simulink model "Simulink_MPC_Main"  (R2023b)
settings: Solver=ode1  StartTime=0.0  StopTime=100  FixedStep=SampleTime  MaxStep=0.01  RelTol=1e-3  EnableMultiTasking=on
values from neighbouring files (symbols this model uses):
  Delay = 3    [Prepare_MPC_005.m]
  FilterDer0 = [8.542800360484532896e-02 ... (first row only)    [Prepare_MPC_005.m]
  FilterDer1 = [2.939212680227305530e+00 ... (first row only)    [Prepare_MPC_005.m]
  SampleTime = 0.05    [Prepare_MPC_005.m]
undefined symbols (not defined in the file or in its folder): GetPosition, length_trajectory_s, poly_approx_trajectory, UpdateBoard
libraries: sldrtlib x1
(part 1 of 2)
settings Model: Creator=jgillis  LastModifiedBy=heib
settings SolverCC: ConcurrentTasks=on  AlgebraicLoopSolver=TrustRegion  PositivePriorityOrder=on  AutoInsertRateTranBlk=on
settings DataIOCC: LimitDataPoints=on  SaveFormat=Array  ReturnWorkspaceOutputs=off
settings OptimizationCC: BlockReduction=off  OptimizeBlockIOStorage=off
settings DebuggingCC: SolverPrmCheckMsg=warning  TasksWithSamePriorityMsg=none  UnconnectedInputMsg=warning  UnconnectedOutputMsg=warning  UnconnectedLineMsg=warning  SFUnexpectedBacktrackingDiag=warning  SFNoUnconditionalDefaultTransitionDiag=warning  SFExecutionAtInitializationDiag=none  ArithmeticOperatorsInVariantConditions=warning
settings HardwareCC: ProdBitPerLong=64  ProdHWDeviceType=Intel->x86-64 (Linux 64)
settings ModelReferenceCC: EnableRefExpFcnMdlSchedulingChecks=on  PropagateSignalLabelsOutOfModel=off
settings SFSimCC: SimUseLocalCustomCode=off  CustomCodeUndefinedFunction=UseInterfaceOnly
settings RTWCC: Description=Simulink Desktop Real-Time  SystemTargetFile=sldrt.tlc  TemplateMakefile=sldrt.tmf  RTWUseLocalCustomCode=off  CustomLibrary=Casadi\casadi.lib  BuildConfiguration=Faster Runs  RTWCompilerOptimization=on
settings CodeAppCC: MaxIdLength=95  StateflowObjectComments=on
settings SimulinkDesktopRealTimeCC: TargetLibSuffix=_sldrt.a  TargetPreCompLibLocation=/home/heib/Documents/Matlab23b/toolbox/sldrt/lib/glnxa64
settings ConfigComp: CovMetricSettings=dw  CovSaveCumulativeToWorkspaceVar=on  CovSaveSingleToWorkspaceVar=on  CovExternalEMLEnable=off  CovSFcnEnable=off

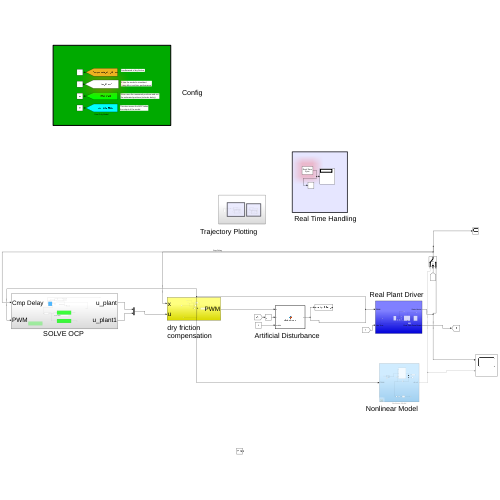
[thumbnail: Simulink's stored preview of the top-level diagram]
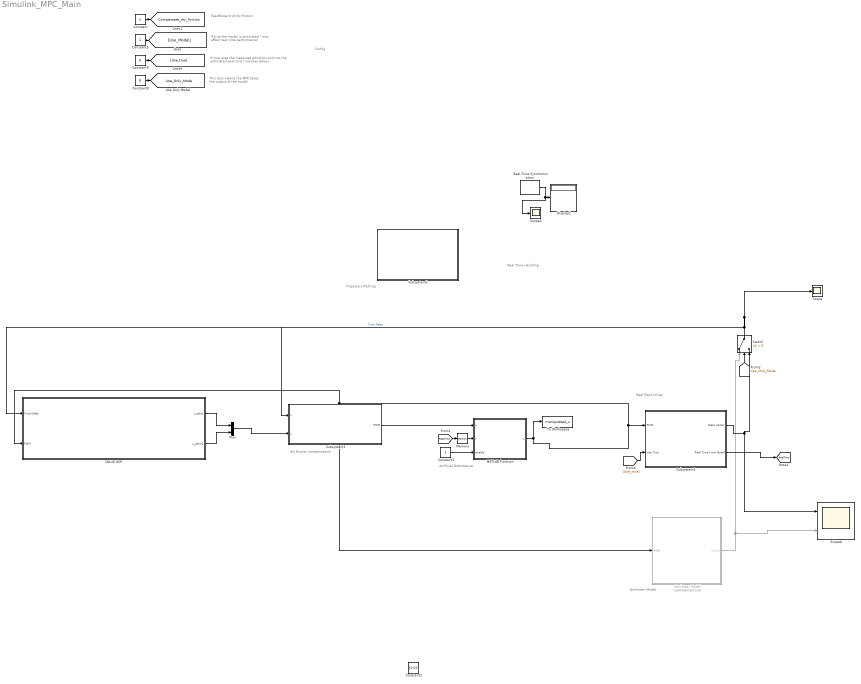
== system Simulink_MPC_Main ==
  note: dry friction compensation
  note: This also means the MPC takes
      | the output of the model
  note: If true the model is simulated
      | ! may affect real time performance!
  note: If true uses the messured positions and not
      | the estimated positions (includes delay).
  note: Feedforward of dry friction
  note: Nonlinear Model
  note: Real Plant Driver
  note: Real Time Handling
  note: Trajectory Plotting
  note: Config
  note: Artificial Disturbance
  Constant : Constant
  Constant1 : Constant
  Constant2 : Constant  Value=[0 0]'
  Constant5 : Constant
  Constant8 : Constant  Value=0
  Constant9 : Constant  Value=0
  Display2 : Display
  MATLAB Function : MATLAB Function  TreatAsAtomicUnit=on
  Memory : Memory
  Mux : Mux  Inputs=2
  Nonlinear Model : Subsystem  Commented=on
  Real-Time Synchronization : sldrtlib/Real-Time Synchronization  SampleTime=SampleTime  MaxMissedTicks=200  ShowMissedTicks=on  YieldWhenWaiting=off
  "SOLVE OCP " : Subsystem
  Scope : Scope
  Scope3 : Scope
  Scope6 : Scope  NumInputPorts=2
  Subsystem1 : Subsystem
  Subsystem2 : Subsystem
  Subsystem3 : Subsystem
  Switch : Switch  Criteria=u2 > Threshold  SaturateOnIntegerOverflow=off  InputSameDT=off
  To Workspace : ToWorkspace  VariableName=manipulated_u  SaveFormat=Timeseries  SampleTime=-1
  tag scope: Compensate_dry_friction=global, RealTime=global, Use_Only_Mode=global
  wires:
  Real-Time Synchronization/1 -> Scope3/1, Display2/1
  MATLAB Function/1(u) -> To Workspace/1, Nonlinear Model/1(PWM), "SOLVE OCP "/2(PWM), Subsystem1/1(PWM)
  Constant8/1 -> [Use_Only_Mode]
  Constant9/1 -> [Use_true]
  Constant5/1 -> [Use_Model]
  Constant/1 -> [Compensate_dry_friction]
  [Use_Only_Mode] -> Switch/2
  Nonlinear Model/1(x0 z-1) -> Scope6/2, Switch/1
  [Use_true] -> Subsystem1/2(Use True)
  Switch/1 -> Scope/1, "SOLVE OCP "/1(Cmp Delay), Subsystem3/1(x)  "Cmp Delay"
  Subsystem1/2(Real Time From Board) -> [RealTime]
  "SOLVE OCP "/1(u_plant) -> Mux/1
  "SOLVE OCP "/2(u_plant1) -> Mux/2
  Subsystem1/1(State Vector) -> Switch/3, Scope6/1
  Mux/1 -> Subsystem3/2(u)
  Subsystem3/1(PWM) -> MATLAB Function/1("u ")
  [RealTime] -> Memory/1
  Memory/1 -> MATLAB Function/2(t)
  Constant1/1 -> MATLAB Function/3(enable)

== system Simulink_MPC_Main/Nonlinear Model ==
  PWM : Inport
  Constant : Constant  Value=0
  Constant1 : Constant  Value=SampleTime
  Demux : Demux  Outputs=2
  MATLAB Function3 : MATLAB Function  TreatAsAtomicUnit=on
  MATLAB Function4 : MATLAB Function  TreatAsAtomicUnit=on
  Memory : Memory  InitialCondition=[GetPosition;zeros(5,1)]'  InheritSampleTime=on
  Memory1 : Memory  InitialCondition=[GetPosition;zeros(5,1)]'  InheritSampleTime=on
  Memory2 : Memory  InitialCondition=[GetPosition;zeros(5,1)]'  InheritSampleTime=on
  Mux : Mux  Inputs=3
  Scope2 : Scope
  To Workspace2 : ToWorkspace  VariableName=Rk4_results  SaveFormat=Timeseries  SampleTime=-1
  x0 z-1 : Outport
  wires:
  MATLAB Function4/1(x_end) -> To Workspace2/1, Memory/1, Scope2/1
  Memory/1 -> Memory1/1, MATLAB Function4/1(x_in)
  PWM/1 -> Demux/1
  Demux/1 -> Mux/1
  Demux/2 -> Mux/2
  Constant/1 -> Mux/3
  Mux/1 -> MATLAB Function4/2(PWM)
  Memory1/1 -> Memory2/1
  Memory2/1 -> MATLAB Function3/1(x)
  Constant1/1 -> MATLAB Function4/3(SampleTime)
  MATLAB Function3/1(current) -> x0 z-1/1

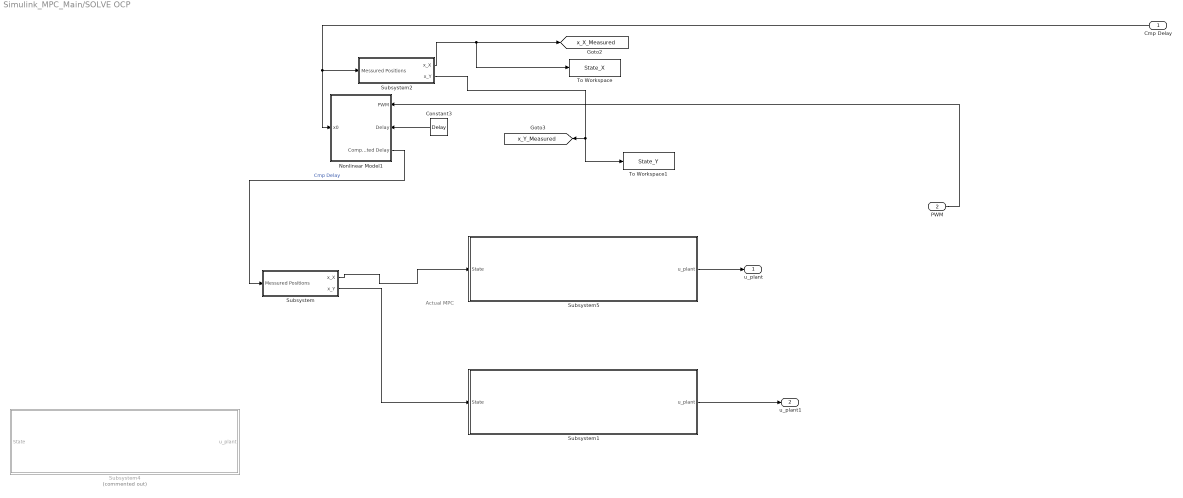
== system Simulink_MPC_Main/SOLVE OCP  ==
  note: Actual MPC
  Cmp Delay : Inport
  PWM : Inport  Port=2
  Constant3 : Constant  Value=Delay
  Nonlinear Model1 : Subsystem
      settings: PortSchema="{\"entries\":[{\"content\":{\"sides\":[{\"content\":{\"connectorIds\":[\"In1\"]},\"type\":\"ConnectorPlacement.EquallySpacedRectSide\",\"uuid\":\"38cfd3d7-56a6-4f45-9bca-759458190eeb\"},{\"content\":{\"connectorIds\":[\"In2\",\"In3\",\"Out1\"],\"side\":\"RIGHT\"},\"type\":\"ConnectorPlacement.EquallySpacedRectSide\",\"uuid\":\"8f579a40-73f0-4433-ae4d-9a35b6fc4d2d\"},{\"content\":{\"side\":\"TOP\"},\"type\":\"ConnectorPlacement.EquallySpacedRectSide\",\"uuid\":\"6933b4ac-f36e-403d-9ee4-935888590ea9\"}]},\"type\":\"ConnectorPlacement.EquallySpacedConnector\",\"uuid\":\"01f2f68f-8bb5-4722-9573-e5e42a50f642\"}],\"packageUris\":[\"http://schema.mathworks.com/mf0/Connector/R2020b\"],\"version\":\"1.0\"}"
  Subsystem : Subsystem
  Subsystem1 : Subsystem
  Subsystem2 : Subsystem
  Subsystem4 : Subsystem  Commented=on
  Subsystem5 : Subsystem
  To Workspace : ToWorkspace  VariableName=State_X  SaveFormat=Timeseries  SampleTime=-1
  To Workspace1 : ToWorkspace  VariableName=State_Y  SaveFormat=Timeseries  SampleTime=-1
  u_plant : Outport
  u_plant1 : Outport  Port=2
  tag scope: x_X_Measured=global, x_Y_Measured=global
  wires:
  Nonlinear Model1/1(Compensated Delay) -> Subsystem/1(Messured Positions)  "Cmp Delay"
  Cmp Delay/1 -> Subsystem2/1(Messured Positions), Nonlinear Model1/1(x0)
  Constant3/1 -> Nonlinear Model1/3(Delay)
  Subsystem1/1(u_plant) -> u_plant1/1
  PWM/1 -> Nonlinear Model1/2(PWM)
  Subsystem5/1(u_plant) -> u_plant/1
  Subsystem/1(x_X) -> Subsystem5/1(State)
  Subsystem/2(x_Y) -> Subsystem1/1(State)
  Subsystem2/1(x_X) -> To Workspace/1, [x_X_Measured]
  Subsystem2/2(x_Y) -> To Workspace1/1, [x_Y_Measured]

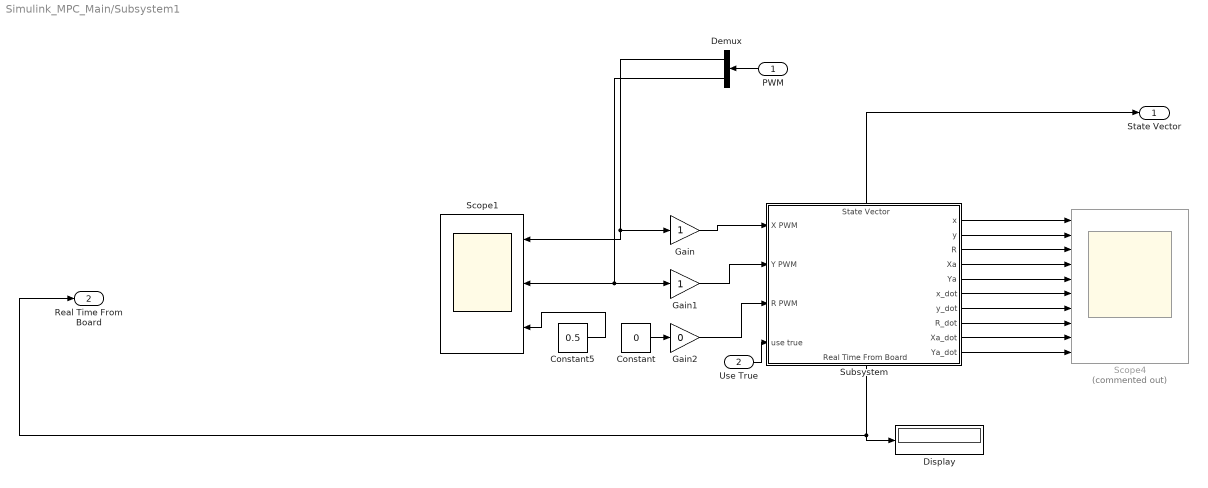
== system Simulink_MPC_Main/Subsystem1 ==
  PWM : Inport
  Use True : Inport  Port=2
  Constant : Constant  Value=0
  Constant5 : Constant  Value=0.5
  Demux : Demux  Outputs=2
  Display : Display
  Gain : Gain
  Gain1 : Gain
  Gain2 : Gain  Gain=0
  Scope1 : Scope  NumInputPorts=3
  Scope4 : Scope  Commented=on  NumInputPorts=10
  Subsystem : Subsystem  StopFcn=UpdateBoard([0 0 0])
      settings: PortSchema="{\"entries\":[{\"content\":{\"sides\":[{\"content\":{\"connectorIds\":[\"In1\",\"In2\",\"In3\",\"In4\"]},\"type\":\"ConnectorPlacement.EquallySpacedRectSide\",\"uuid\":\"9c191be3-a45d-4bde-908f-a93b32fc7100\"},{\"content\":{\"connectorIds\":[\"Out1\",\"Out2\",\"Out3\",\"Out4\",\"Out5\",\"Out6\",\"Out7\",\"Out8\",\"Out9\",\"Out10\"],\"side\":\"RIGHT\"},\"type\":\"ConnectorPlacement.EquallySpacedRectSide\",\"uuid\":\"786ae7fd-3fdd-4e4f-b32e-e8a30c9c90df\"},{\"content\":{\"connectorIds\":[\"Out12\"],\"side\":\"TOP\"},\"type\":\"ConnectorPlacement.EquallySpacedRectSide\",\"uuid\":\"660763ff-34dc-4c5b-8e93-3606a4818ae8\"},{\"content\":{\"connectorIds\":[\"Out11\"],\"side\":\"BOTTOM\"},\"type\":\"ConnectorPlacement.EquallySpacedRectSide\",\"uuid\":\"dc7e5dc1-ad21-4d2b-aff3-6d4be469e1a4\"}]},\"type\":\"ConnectorPlacement.EquallySpacedConnector\",\"uuid\":\"7e886ff6-44b8-4e6d-bf22-6606d53ee007\"}],\"packageUris\":[\"http://schema.mathworks.com/mf0/Connector/R2020b\"],\"version\":\"1.0\"}"
  State Vector : Outport
  Real Time From Board : Outport  Port=2
  wires:
  Subsystem/4(Xa) -> Scope4/4
  Subsystem/1(x) -> Scope4/1
  Subsystem/9(Xa_dot) -> Scope4/9
  Subsystem/10(Ya_dot) -> Scope4/10
  Subsystem/3(R) -> Scope4/3
  Subsystem/8(R_dot) -> Scope4/8
  Subsystem/7(y_dot) -> Scope4/7
  Subsystem/11(Real Time From Board) -> Real Time From Board/1, Display/1
  Subsystem/5(Ya) -> Scope4/5
  Subsystem/12(State Vector) -> State Vector/1
  Constant5/1 -> Scope1/3
  Gain/1 -> Subsystem/1(X PWM)
  Subsystem/2(y) -> Scope4/2
  Gain2/1 -> Subsystem/3(R PWM)
  Subsystem/6(x_dot) -> Scope4/6
  Demux/1 -> Scope1/1, Gain/1
  Demux/2 -> Gain1/1, Scope1/2
  Constant/1 -> Gain2/1
  Gain1/1 -> Subsystem/2(Y PWM)
  PWM/1 -> Demux/1
  Use True/1 -> Subsystem/4(use true)

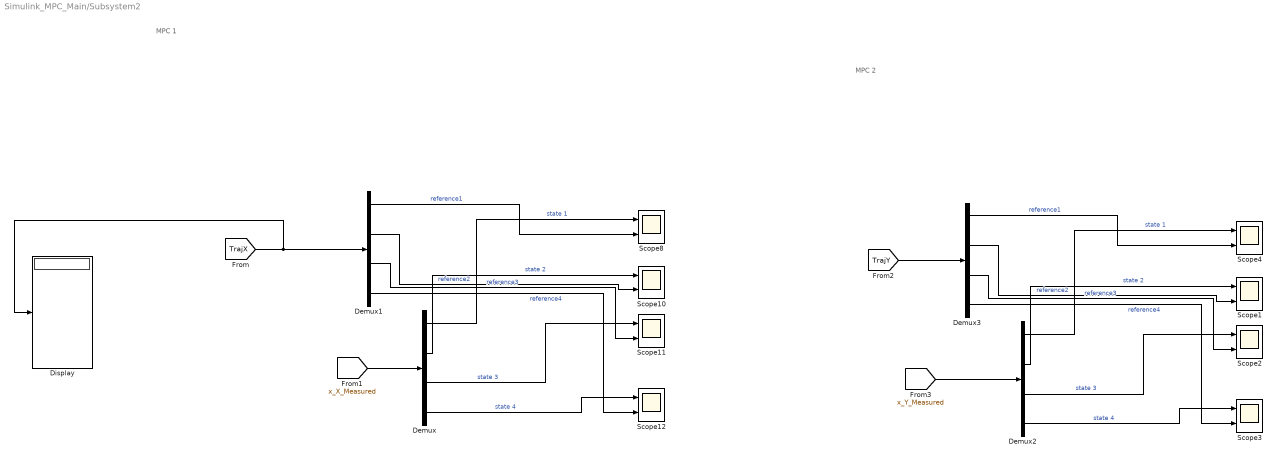
== system Simulink_MPC_Main/Subsystem2 ==
  note: MPC 1
  note: MPC 2
  Demux{,1..3} (4 alike) : Demux
  Display : Display
  Scope{1..4,8,10..12} (8 alike) : Scope  NumInputPorts=2
  wires:
  [x_X_Measured] -> Demux/1
  Demux/1 -> Scope8/1  "state 1"
  Demux/2 -> Scope10/1  "state 2"
  Demux/3 -> Scope11/1  "state 3"
  Demux/4 -> Scope12/1  "state 4"
  Demux1/4 -> Scope12/2  "reference4"
  Demux1/3 -> Scope11/2  "reference3"
  Demux1/2 -> Scope10/2  "reference2"
  Demux1/1 -> Scope8/2  "reference1"
  Demux2/4 -> Scope3/1  "state 4"
  [x_Y_Measured] -> Demux2/1
  Demux2/2 -> Scope1/1  "state 2"
  Demux3/3 -> Scope2/2  "reference3"
  Demux3/2 -> Scope1/2  "reference2"
  Demux3/4 -> Scope3/2  "reference4"
  Demux2/3 -> Scope2/1  "state 3"
  Demux2/1 -> Scope4/1  "state 1"
  Demux3/1 -> Scope4/2  "reference1"
  [TrajX] -> Demux1/1, Display/1
  [TrajY] -> Demux3/1

== system Simulink_MPC_Main/Subsystem3 ==
  x : Inport
  u : Inport  Port=2
  Scope : Scope  NumInputPorts=2
  Switch : Switch  Criteria=u2 > Threshold  SaturateOnIntegerOverflow=off  InputSameDT=off
  To Workspace3 : ToWorkspace  VariableName=PWM_toPlant  SaveFormat=Timeseries  SampleTime=-1
  dry_friction_compensation : MATLAB Function  TreatAsAtomicUnit=on
  PWM : Outport
  wires:
  x/1 -> dry_friction_compensation/1(x)
  dry_friction_compensation/1(u_compensated) -> Switch/1
  u/1 -> Scope/1, dry_friction_compensation/2(u), Switch/3
  Switch/1 -> Scope/2, To Workspace3/1, PWM/1
  [Compensate_dry_friction] -> Switch/2

== system Simulink_MPC_Main/SOLVE OCP /Nonlinear Model1 ==
  x0 : Inport
  PWM : Inport  Port=2
  Delay : Inport  Port=3
  Constant : Constant  Value=0
  Constant1 : Constant  Value=SampleTime
  Demux : Demux  Outputs=2
  MATLAB Function : MATLAB Function  TreatAsAtomicUnit=on
  MATLAB Function11 : MATLAB Function  TreatAsAtomicUnit=on
  MATLAB Function4 : MATLAB Function  TreatAsAtomicUnit=on
  Mux : Mux  Inputs=3
  Scope : Scope  NumInputPorts=2
  Compensated Delay : Outport
  wires:
  x0/1 -> Scope/2, MATLAB Function4/1(x_in)  "measured"
  PWM/1 -> Demux/1
  Demux/1 -> Mux/1
  Demux/2 -> Mux/2
  Constant/1 -> Mux/3
  Constant1/1 -> MATLAB Function4/3(SampleTime)
  Delay/1 -> MATLAB Function4/4(Delay)
  MATLAB Function4/1(x_end) -> Scope/1, MATLAB Function/1(x)
  Mux/1 -> MATLAB Function11/1(u)
  MATLAB Function11/1(y) -> MATLAB Function4/2(PWM)
  MATLAB Function/1(x_bound) -> Compensated Delay/1

== system Simulink_MPC_Main/SOLVE OCP /Subsystem ==
  note: Integrator Logic
      | Gemessene Position kommt von Plant
      | und Integral anteil fehler kommt con MPC
  Messured Positions : Inport
  Delete L : MATLAB Function  TreatAsAtomicUnit=on
  MATLAB Function10 : MATLAB Function  TreatAsAtomicUnit=on
  Scope : Scope  Commented=on
  To Workspace5 : ToWorkspace  VariableName=x0_out  SaveFormat=Structure With Time  SampleTime=-1
  x_X : Outport
  x_Y : Outport  Port=2
  wires:
  MATLAB Function10/1(x_X) -> x_X/1, To Workspace5/1
  Messured Positions/1 -> Delete L/1(x10)
  Delete L/1(x_8) -> Scope/1, MATLAB Function10/1(x_18)
  MATLAB Function10/2(x_Y) -> x_Y/1

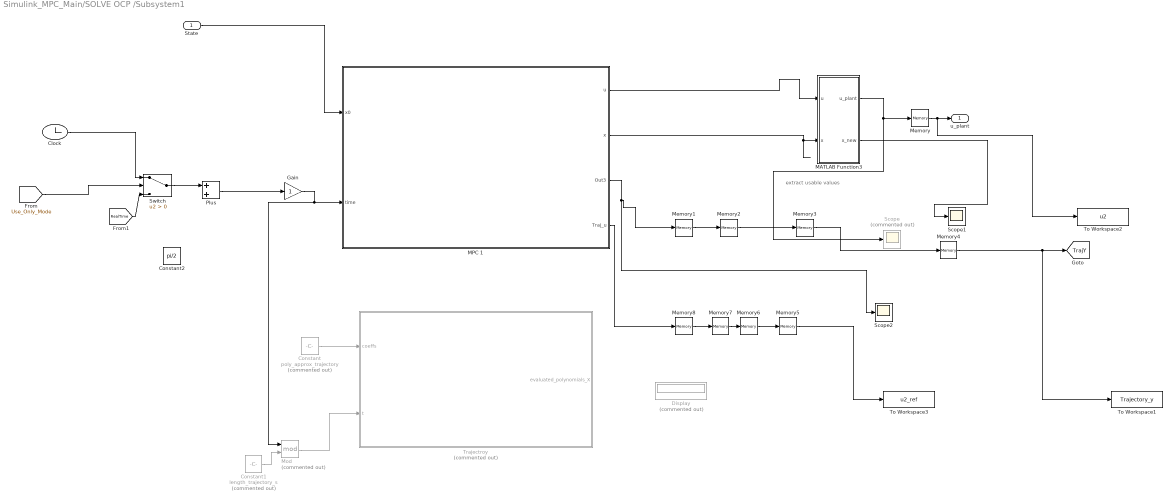
== system Simulink_MPC_Main/SOLVE OCP /Subsystem1 ==
  note: extract usable values
  State : Inport
  Clock : Clock
  Constant : Constant  Commented=on  Value=poly_approx_trajectory
  Constant1 : Constant  Commented=on  Value=length_trajectory_s
  Constant2 : Constant  Value=pi/2
  Display : Display  Commented=on
  Gain : Gain
  MATLAB Function3 : MATLAB Function  TreatAsAtomicUnit=on
  MPC 1 : Subsystem
  Memory{,1..8} (9 alike) : Memory
  Mod : Math  Commented=on  Operator=mod
  Plus : Sum
  Scope : Scope  Commented=on
  Scope1 : Scope
  Scope2 : Scope
  Switch : Switch  Criteria=u2 > Threshold  SaturateOnIntegerOverflow=off  InputSameDT=off
  To Workspace1 : ToWorkspace  VariableName=Trajectory_y  SaveFormat=Timeseries  SampleTime=-1
  To Workspace2 : ToWorkspace  VariableName=u2  SaveFormat=Timeseries  SampleTime=-1
  To Workspace3 : ToWorkspace  VariableName=u2_ref  SaveFormat=Timeseries  SampleTime=-1
  Trajectroy : MATLAB Function  Commented=on  TreatAsAtomicUnit=on
  u_plant : Outport
  tag scope: TrajY=global
  wires:
  MPC 1/2(x) -> MATLAB Function3/2(x)
  MPC 1/1(u) -> MATLAB Function3/1(u)
  Switch/1 -> Plus/1
  MATLAB Function3/1(u_plant) -> Scope/1, Memory/1
  Gain/1 -> MPC 1/2(time), Mod/1
  State/1 -> MPC 1/1(x0)
  Memory/1 -> To Workspace2/1, u_plant/1
  [Use_Only_Mode] -> Switch/2
  Clock/1 -> Switch/1
  [RealTime] -> Switch/3
  MATLAB Function3/2(x_new) -> Scope1/1
  Constant/1 -> Trajectroy/1(coeffs)
  Constant1/1 -> Mod/2
  Mod/1 -> Trajectroy/2(t)
  MPC 1/4(Traj_u) -> Memory8/1
  Plus/1 -> Gain/1
  Memory1/1 -> Memory2/1
  Memory2/1 -> Memory3/1
  Memory3/1 -> Memory4/1
  Memory4/1 -> To Workspace1/1, [TrajY]
  MPC 1/3(Out3) -> Memory1/1, Scope2/1
  Memory7/1 -> Memory6/1
  Memory5/1 -> To Workspace3/1
  Memory8/1 -> Memory7/1
  Memory6/1 -> Memory5/1

== system Simulink_MPC_Main/SOLVE OCP /Subsystem2 ==
  note: Integrator Logic
      | Gemessene Position kommt von Plant
      | und Integral anteil fehler kommt con MPC
  Messured Positions : Inport
  Delete L : MATLAB Function  TreatAsAtomicUnit=on
  MATLAB Function10 : MATLAB Function  TreatAsAtomicUnit=on
  Scope : Scope  Commented=on
  x_X : Outport
  x_Y : Outport  Port=2
  wires:
  MATLAB Function10/1(x_X) -> x_X/1
  Delete L/1(x_8) -> Scope/1, MATLAB Function10/1(x_18)
  MATLAB Function10/2(x_Y) -> x_Y/1
  Messured Positions/1 -> Delete L/1(x10)

== system Simulink_MPC_Main/SOLVE OCP /Subsystem4 ==
  note: extract usable values
  State : Inport
  Clock : Clock
  Constant : Constant  Value=3*pi/2
  Display : Display
  Gain : Gain
  MATLAB Function3 : MATLAB Function  TreatAsAtomicUnit=on
  MPC 1 : Subsystem
  Memory : Memory
  Plus : Sum
  Scope : Scope
  Scope1 : Scope
  u_plant : Outport
  tag scope: TrajY=global
  wires:
  MATLAB Function3/1(u_plant) -> Memory/1, Scope/1
  MPC 1/2(x) -> MATLAB Function3/2(x)
  MPC 1/1(u) -> MATLAB Function3/1(u), Display/1
  Clock/1 -> Plus/1
  Memory/1 -> u_plant/1
  MPC 1/3(Out3) -> [TrajY]
  Gain/1 -> MPC 1/2(time)
  State/1 -> Scope1/1, MPC 1/1(x0)
  Constant/1 -> Plus/2
  Plus/1 -> Gain/1

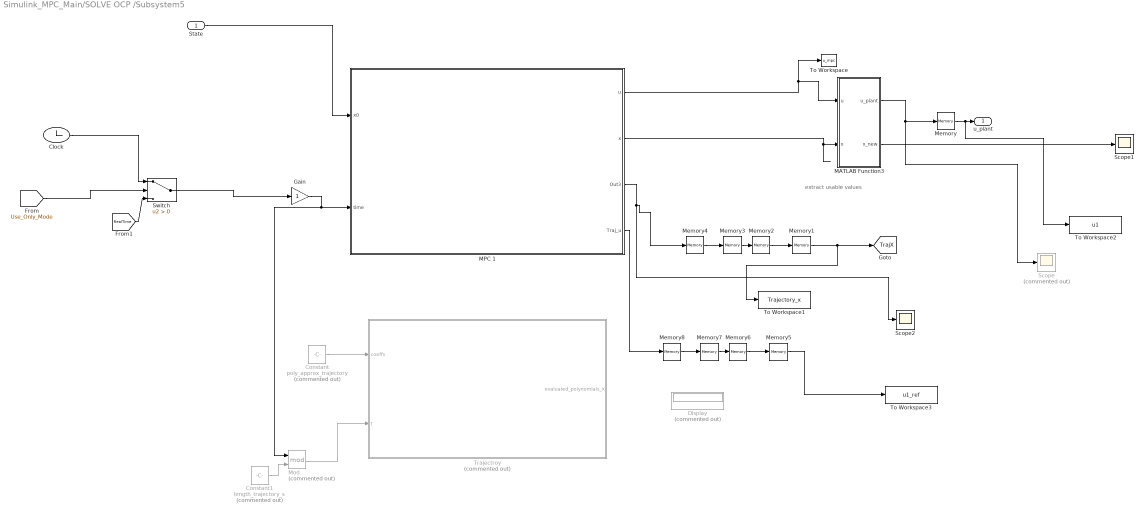
== system Simulink_MPC_Main/SOLVE OCP /Subsystem5 ==
  note: extract usable values
  State : Inport
  Clock : Clock
  Constant : Constant  Commented=on  Value=poly_approx_trajectory
  Constant1 : Constant  Commented=on  Value=length_trajectory_s
  Display : Display  Commented=on
  Gain : Gain
  MATLAB Function3 : MATLAB Function  TreatAsAtomicUnit=on
  MPC 1 : Subsystem
  Memory{,1..8} (9 alike) : Memory
  Mod : Math  Commented=on  Operator=mod
  Scope : Scope  Commented=on
  Scope1 : Scope
  Scope2 : Scope
  Switch : Switch  Criteria=u2 > Threshold  SaturateOnIntegerOverflow=off  InputSameDT=off
  To Workspace : ToWorkspace  VariableName=u_mpc  SaveFormat=Timeseries  SampleTime=-1
  To Workspace1 : ToWorkspace  VariableName=Trajectory_x  SaveFormat=Timeseries  SampleTime=-1
  To Workspace2 : ToWorkspace  VariableName=u1  SaveFormat=Timeseries  SampleTime=-1
  To Workspace3 : ToWorkspace  VariableName=u1_ref  SaveFormat=Timeseries  SampleTime=-1
  Trajectroy : MATLAB Function  Commented=on  TreatAsAtomicUnit=on
  u_plant : Outport
  tag scope: TrajX=global
  wires:
  MPC 1/2(x) -> MATLAB Function3/2(x)
  MPC 1/1(u) -> MATLAB Function3/1(u), To Workspace/1
  Switch/1 -> Gain/1
  Gain/1 -> MPC 1/2(time), Mod/1
  State/1 -> MPC 1/1(x0)
  MATLAB Function3/1(u_plant) -> Memory/1, Scope/1
  [Use_Only_Mode] -> Switch/2
  Clock/1 -> Switch/1
  [RealTime] -> Switch/3
  MPC 1/3(Out3) -> Memory4/1, Scope2/1
  Constant/1 -> Trajectroy/1(coeffs)
  Constant1/1 -> Mod/2
  Mod/1 -> Trajectroy/2(t)
  MATLAB Function3/2(x_new) -> Scope1/1
  Memory/1 -> To Workspace2/1, u_plant/1
  MPC 1/4(Traj_u) -> Memory8/1
  Memory1/1 -> To Workspace1/1, [TrajX]
  Memory2/1 -> Memory1/1
  Memory3/1 -> Memory2/1
  Memory4/1 -> Memory3/1
  Memory7/1 -> Memory6/1
  Memory8/1 -> Memory7/1
  Memory5/1 -> To Workspace3/1
  Memory6/1 -> Memory5/1

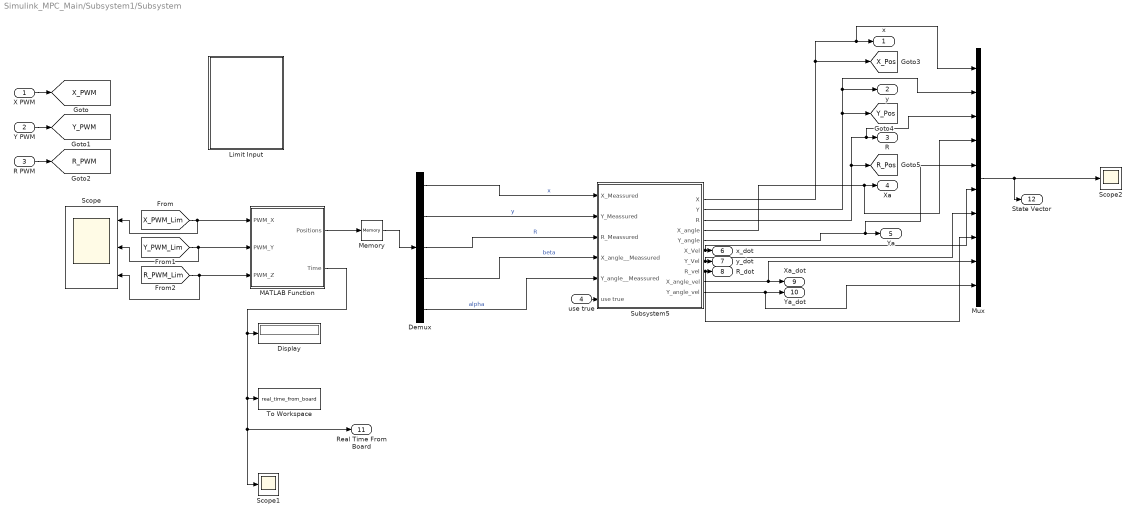
== system Simulink_MPC_Main/Subsystem1/Subsystem ==
  X PWM : Inport
  Y PWM : Inport  Port=2
  R PWM : Inport  Port=3
  use true : Inport  Port=4
  Demux : Demux  Outputs=5
  Display : Display
  Limit Input : Subsystem
  MATLAB Function : MATLAB Function  TreatAsAtomicUnit=on
  Memory : Memory  InitialCondition=GetPosition'  InheritSampleTime=on
  Mux : Mux  Inputs=10
  Scope : Scope  NumInputPorts=3
  Scope1 : Scope
  Scope2 : Scope
  Subsystem5 : Subsystem
  To Workspace : ToWorkspace  VariableName=real_time_from_board  SaveFormat=Structure With Time  SampleTime=-1
  x : Outport
  y : Outport  Port=2
  R : Outport  Port=3
  Xa : Outport  Port=4
  Ya : Outport  Port=5
  x_dot : Outport  Port=6
  y_dot : Outport  Port=7
  R_dot : Outport  Port=8
  Xa_dot : Outport  Port=9
  Ya_dot : Outport  Port=10
  Real Time From Board : Outport  Port=11
  State Vector : Outport  Port=12
  tag scope: R_PWM=global, R_Pos=global, X_PWM=global, X_Pos=global, Y_PWM=global, Y_Pos=global
  wires:
  MATLAB Function/1(Positions) -> Memory/1
  [X_PWM_Lim] -> Scope/1, MATLAB Function/1(PWM_X)
  [Y_PWM_Lim] -> Scope/2, MATLAB Function/2(PWM_Y)
  Memory/1 -> Demux/1
  Subsystem5/1(X) -> Mux/1, x/1, [X_Pos]
  Subsystem5/3(R) -> Mux/3, R/1, [R_Pos]
  Subsystem5/4(X_angle) -> Mux/4, Xa/1
  Subsystem5/5(Y_angle) -> Mux/5, Ya/1
  R PWM/1 -> [R_PWM]
  Y PWM/1 -> [Y_PWM]
  X PWM/1 -> [X_PWM]
  [R_PWM_Lim] -> Scope/3, MATLAB Function/3(PWM_Z)
  Demux/1 -> Subsystem5/1(X_Meassured)  "x"
  Demux/2 -> Subsystem5/2(Y_Meassured)  "y"
  Demux/3 -> Subsystem5/3(R_Meassured)  "R"
  Demux/4 -> Subsystem5/4(X_angle__Meassured)  "beta"
  Demux/5 -> Subsystem5/5(Y_angle__Meassured)  "alpha"
  Subsystem5/6(X_Vel) -> Mux/6, x_dot/1
  Subsystem5/7(Y_Vel) -> Mux/7, y_dot/1
  Subsystem5/8(R_vel) -> Mux/8, R_dot/1
  Subsystem5/9(X_angle_vel) -> Mux/9, Xa_dot/1
  Subsystem5/10(Y_angle_vel) -> Mux/10, Ya_dot/1
  MATLAB Function/2(Time) -> To Workspace/1, Real Time From Board/1, Scope1/1, Display/1
  Subsystem5/2(Y) -> Mux/2, y/1, [Y_Pos]
  Mux/1 -> State Vector/1, Scope2/1
  use true/1 -> Subsystem5/6(use true)

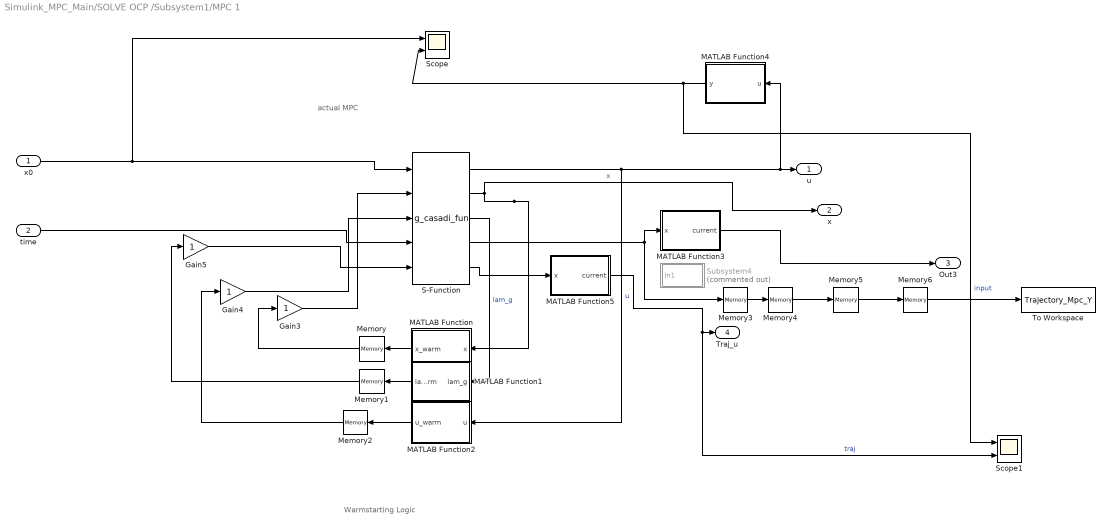
== system Simulink_MPC_Main/SOLVE OCP /Subsystem1/MPC 1 ==
  note: actual MPC
  note: Warmstarting Logic
  x0 : Inport
  time : Inport  Port=2
  Gain3 : Gain
  Gain4 : Gain
  Gain5 : Gain
  MATLAB Function : MATLAB Function  TreatAsAtomicUnit=on
  MATLAB Function1 : MATLAB Function  TreatAsAtomicUnit=on
  MATLAB Function2 : MATLAB Function  TreatAsAtomicUnit=on
  MATLAB Function3 : MATLAB Function  TreatAsAtomicUnit=on
  MATLAB Function4 : MATLAB Function  TreatAsAtomicUnit=on
  MATLAB Function5 : MATLAB Function  TreatAsAtomicUnit=on
  Memory{,1..6} (7 alike) : Memory
  S-Function : S-Function  FunctionName=g_casadi_fun  Parameters='g.casadi', 'g'  SFunctionDeploymentMode=off  EnableBusSupport=off
  Scope : Scope  NumInputPorts=2
  Scope1 : Scope  NumInputPorts=2
  Subsystem4 : Subsystem  Commented=on
  To Workspace : ToWorkspace  VariableName=Trajectory_Mpc_Y  SaveFormat=Timeseries  SampleTime=-1
  u : Outport
  x : Outport  Port=2
  Out3 : Outport  Port=3
  Traj_u : Outport  Port=4
  wires:
  Gain3/1 -> S-Function/2
  Gain4/1 -> S-Function/3
  Memory1/1 -> Gain5/1
  ? -> Subsystem4/1(In1)
  MATLAB Function2/1(u_warm) -> Memory2/1
  MATLAB Function1/1(lam_g_warm) -> Memory1/1
  S-Function/2 -> MATLAB Function/1(x), x/1  "x"
  x0/1 -> Scope/1, S-Function/1
  S-Function/1 -> MATLAB Function4/1(u), u/1, MATLAB Function2/1(u)  "u"
  S-Function/3 -> MATLAB Function1/1(lam_g)  "lam_g"
  Memory/1 -> Gain3/1
  Gain5/1 -> S-Function/5
  Memory2/1 -> Gain4/1
  MATLAB Function/1(x_warm) -> Memory/1
  time/1 -> S-Function/4
  S-Function/4 -> MATLAB Function3/1(x), Memory3/1
  MATLAB Function3/1(current) -> Out3/1
  MATLAB Function4/1(y) -> Scope1/1, Scope/2  "input"
  S-Function/5 -> MATLAB Function5/1(x)
  MATLAB Function5/1(current) -> Scope1/2, Traj_u/1  "traj"
  Memory3/1 -> Memory4/1
  Memory4/1 -> Memory5/1
  Memory6/1 -> To Workspace/1
  Memory5/1 -> Memory6/1

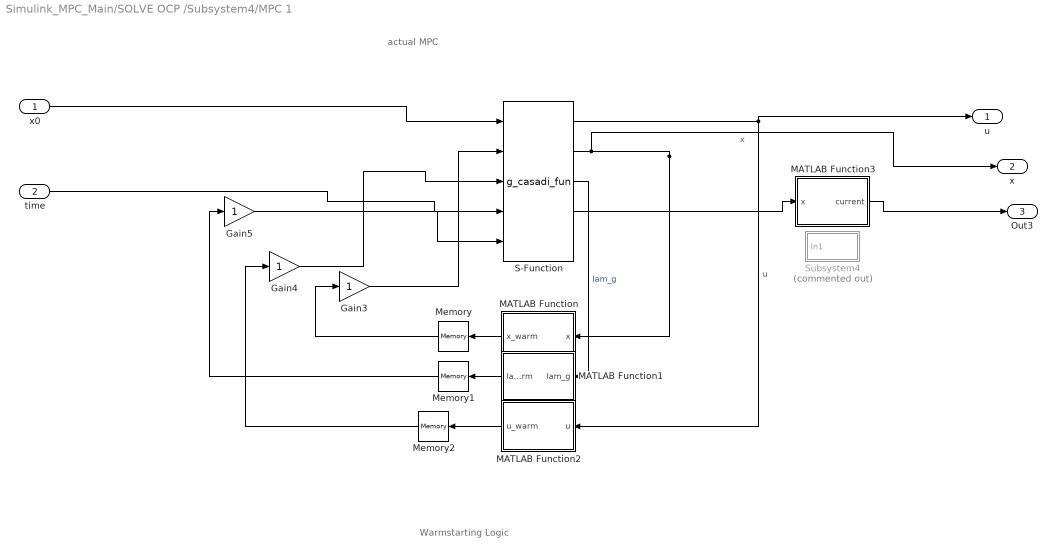
== system Simulink_MPC_Main/SOLVE OCP /Subsystem4/MPC 1 ==
  note: actual MPC
  note: Warmstarting Logic
  x0 : Inport
  time : Inport  Port=2
  Gain3 : Gain
  Gain4 : Gain
  Gain5 : Gain
  MATLAB Function : MATLAB Function  TreatAsAtomicUnit=on
  MATLAB Function1 : MATLAB Function  TreatAsAtomicUnit=on
  MATLAB Function2 : MATLAB Function  TreatAsAtomicUnit=on
  MATLAB Function3 : MATLAB Function  TreatAsAtomicUnit=on
  Memory : Memory
  Memory1 : Memory
  Memory2 : Memory
  S-Function : S-Function  FunctionName=g_casadi_fun  Parameters='g.casadi', 'g'  SFunctionDeploymentMode=off  EnableBusSupport=off
  Subsystem4 : Subsystem  Commented=on
  u : Outport
  x : Outport  Port=2
  Out3 : Outport  Port=3
  wires:
  Gain3/1 -> S-Function/2
  Gain4/1 -> S-Function/3
  Memory1/1 -> Gain5/1
  ? -> Subsystem4/1(In1)
  MATLAB Function2/1(u_warm) -> Memory2/1
  MATLAB Function1/1(lam_g_warm) -> Memory1/1
  S-Function/4 -> MATLAB Function3/1(x)
  S-Function/2 -> MATLAB Function/1(x), x/1  "x"
  x0/1 -> S-Function/1
  S-Function/1 -> u/1, MATLAB Function2/1(u)  "u"
  S-Function/3 -> MATLAB Function1/1(lam_g)  "lam_g"
  Memory/1 -> Gain3/1
  Gain5/1 -> S-Function/5
  Memory2/1 -> Gain4/1
  MATLAB Function/1(x_warm) -> Memory/1
  time/1 -> S-Function/4
  MATLAB Function3/1(current) -> Out3/1

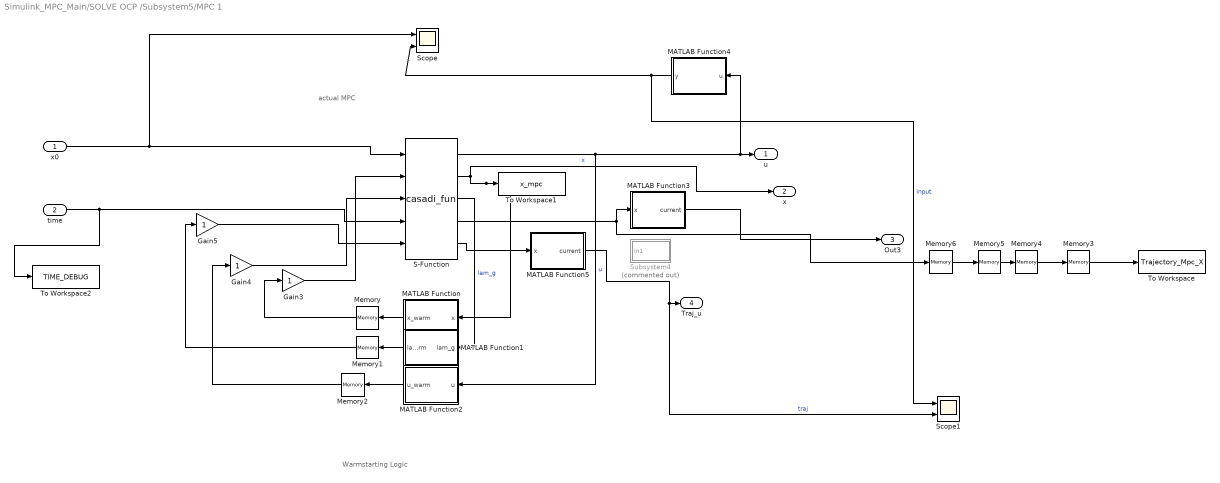
== system Simulink_MPC_Main/SOLVE OCP /Subsystem5/MPC 1 ==
  note: actual MPC
  note: Warmstarting Logic
  x0 : Inport
  time : Inport  Port=2
  Gain3 : Gain
  Gain4 : Gain
  Gain5 : Gain
  MATLAB Function : MATLAB Function  TreatAsAtomicUnit=on
  MATLAB Function1 : MATLAB Function  TreatAsAtomicUnit=on
  MATLAB Function2 : MATLAB Function  TreatAsAtomicUnit=on
  MATLAB Function3 : MATLAB Function  TreatAsAtomicUnit=on
  MATLAB Function4 : MATLAB Function  TreatAsAtomicUnit=on
  MATLAB Function5 : MATLAB Function  TreatAsAtomicUnit=on
  Memory{,1..6} (7 alike) : Memory
  S-Function : S-Function  FunctionName=casadi_fun  Parameters='f.casadi', 'f'  SFunctionDeploymentMode=off  EnableBusSupport=off
  Scope : Scope  NumInputPorts=2
  Scope1 : Scope  NumInputPorts=2
  Subsystem4 : Subsystem  Commented=on
  To Workspace : ToWorkspace  VariableName=Trajectory_Mpc_X  SaveFormat=Timeseries  SampleTime=-1
  To Workspace1 : ToWorkspace  VariableName=x_mpc  SaveFormat=Timeseries  SampleTime=-1
  To Workspace2 : ToWorkspace  VariableName=TIME_DEBUG  SaveFormat=Timeseries  SampleTime=-1
  u : Outport
  x : Outport  Port=2
  Out3 : Outport  Port=3
  Traj_u : Outport  Port=4
  wires:
  Gain3/1 -> S-Function/2
  Gain4/1 -> S-Function/3
  Memory1/1 -> Gain5/1
  ? -> Subsystem4/1(In1)
  MATLAB Function2/1(u_warm) -> Memory2/1
  MATLAB Function1/1(lam_g_warm) -> Memory1/1
  S-Function/2 -> MATLAB Function/1(x), To Workspace1/1, x/1  "x"
  x0/1 -> Scope/1, S-Function/1
  S-Function/1 -> MATLAB Function4/1(u), u/1, MATLAB Function2/1(u)  "u"
  S-Function/3 -> MATLAB Function1/1(lam_g)  "lam_g"
  Memory/1 -> Gain3/1
  Gain5/1 -> S-Function/5
  Memory2/1 -> Gain4/1
  MATLAB Function/1(x_warm) -> Memory/1
  time/1 -> To Workspace2/1, S-Function/4
  S-Function/4 -> MATLAB Function3/1(x), Memory6/1
  MATLAB Function3/1(current) -> Out3/1
  MATLAB Function4/1(y) -> Scope1/1, Scope/2  "input"
  S-Function/5 -> MATLAB Function5/1(x)
  MATLAB Function5/1(current) -> Scope1/2, Traj_u/1  "traj"
  Memory5/1 -> Memory4/1
  Memory3/1 -> To Workspace/1
  Memory4/1 -> Memory3/1
  Memory6/1 -> Memory5/1

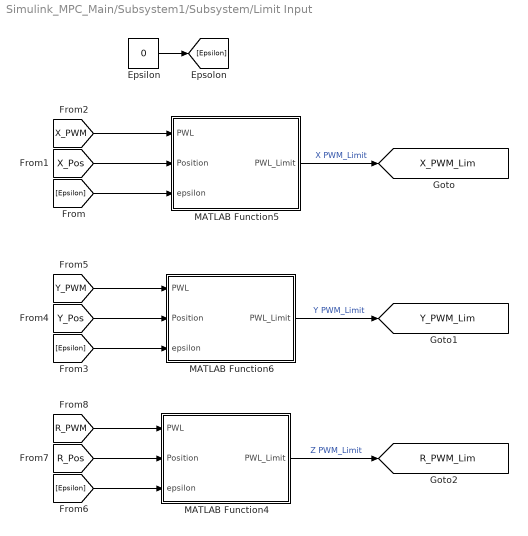
== system Simulink_MPC_Main/Subsystem1/Subsystem/Limit Input ==
  Epsilon : Constant  Value=0
  MATLAB Function4 : MATLAB Function  TreatAsAtomicUnit=on
  MATLAB Function5 : MATLAB Function  TreatAsAtomicUnit=on
  MATLAB Function6 : MATLAB Function  TreatAsAtomicUnit=on
  tag scope: R_PWM_Lim=global, X_PWM_Lim=global, Y_PWM_Lim=global
  wires:
  Epsilon/1 -> [Epsilon]
  [Epsilon] -> MATLAB Function5/3(epsilon)
  [X_Pos] -> MATLAB Function5/2(Position)
  [X_PWM] -> MATLAB Function5/1(PWL)
  MATLAB Function5/1(PWL_Limit) -> [X_PWM_Lim]  "X PWM_Limit"
  [Y_PWM] -> MATLAB Function6/1(PWL)
  [Epsilon] -> MATLAB Function6/3(epsilon)
  [Y_Pos] -> MATLAB Function6/2(Position)
  [R_Pos] -> MATLAB Function4/2(Position)
  [Epsilon] -> MATLAB Function4/3(epsilon)
  [R_PWM] -> MATLAB Function4/1(PWL)
  MATLAB Function4/1(PWL_Limit) -> [R_PWM_Lim]  "Z PWM_Limit"
  MATLAB Function6/1(PWL_Limit) -> [Y_PWM_Lim]  "Y PWM_Limit"

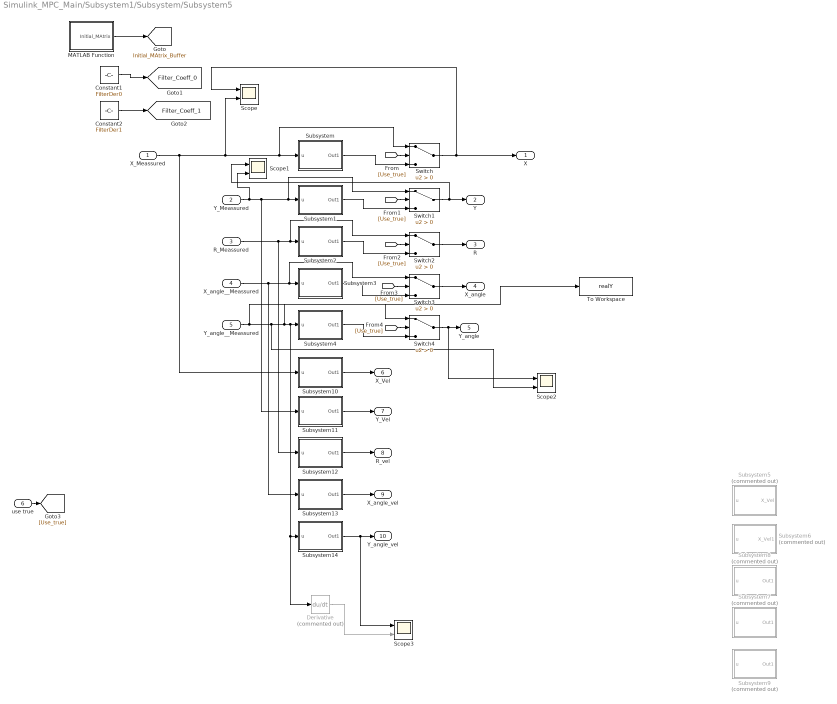
== system Simulink_MPC_Main/Subsystem1/Subsystem/Subsystem5 ==
  X_Meassured : Inport
  Y_Meassured : Inport  Port=2
  R_Meassured : Inport  Port=3
  X_angle__Meassured : Inport  Port=4
  Y_angle__Meassured : Inport  Port=5
  use true : Inport  Port=6
  Constant1 : Constant  Value=FilterDer0
  Constant2 : Constant  Value=FilterDer1
  Derivative : Derivative  Commented=on
  MATLAB Function : MATLAB Function  TreatAsAtomicUnit=on
  Scope{,1..3} (4 alike) : Scope  NumInputPorts=2
  Subsystem : Subsystem
  Subsystem1 : Subsystem
  Subsystem10 : Subsystem
  Subsystem11 : Subsystem
  Subsystem12 : Subsystem
  Subsystem13 : Subsystem
  Subsystem14 : Subsystem
  Subsystem2 : Subsystem
  Subsystem3 : Subsystem
  Subsystem4 : Subsystem
  Subsystem5 : Subsystem  Commented=on
  Subsystem6 : Subsystem  Commented=on
  Subsystem7 : Subsystem  Commented=on
  Subsystem8 : Subsystem  Commented=on
  Subsystem9 : Subsystem  Commented=on
  Switch{,1..4} (5 alike) : Switch  Criteria=u2 > Threshold  SaturateOnIntegerOverflow=off  InputSameDT=off
  To Workspace : ToWorkspace  VariableName=realY  SaveFormat=Timeseries  SampleTime=-1
  X : Outport
  Y : Outport  Port=2
  R : Outport  Port=3
  X_angle : Outport  Port=4
  Y_angle : Outport  Port=5
  X_Vel : Outport  Port=6
  Y_Vel : Outport  Port=7
  R_vel : Outport  Port=8
  X_angle_vel : Outport  Port=9
  Y_angle_vel : Outport  Port=10
  tag scope: Filter_Coeff_0=global, Filter_Coeff_1=global, Initial_MAtrix_Buffer=global
  wires:
  X_angle__Meassured/1 -> Subsystem13/1(u), Subsystem3/1(u), Switch3/1
  R_Meassured/1 -> Subsystem12/1(u), Subsystem2/1(u), Switch2/1
  Y_Meassured/1 -> Scope1/2, Subsystem11/1(u), Subsystem1/1(u), Switch1/1
  X_Meassured/1 -> Subsystem10/1(u), Scope/2, Switch/1, Subsystem/1(u)
  Y_angle__Meassured/1 -> To Workspace/1, Scope2/2, Switch4/1, Subsystem4/1(u), Subsystem14/1(u), Derivative/1
  Subsystem10/1(Out1) -> X_Vel/1
  Subsystem14/1(Out1) -> Scope3/1, Y_angle_vel/1
  Subsystem13/1(Out1) -> X_angle_vel/1
  Subsystem12/1(Out1) -> R_vel/1
  Subsystem11/1(Out1) -> Y_Vel/1
  Subsystem/1(Out1) -> Switch/3
  Switch/1 -> Scope/1, X/1
  [Use_true] -> Switch/2
  [Use_true] -> Switch1/2
  Switch1/1 -> Scope1/1, Y/1
  [Use_true] -> Switch2/2
  [Use_true] -> Switch3/2
  [Use_true] -> Switch4/2
  Switch2/1 -> R/1
  Switch3/1 -> X_angle/1
  Switch4/1 -> Scope2/1, Y_angle/1
  Subsystem1/1(Out1) -> Switch1/3
  Subsystem2/1(Out1) -> Switch2/3
  Subsystem3/1(Out1) -> Switch3/3
  Subsystem4/1(Out1) -> Switch4/3
  MATLAB Function/1(Initial_MAtrix) -> [Initial_MAtrix_Buffer]
  Constant1/1 -> [Filter_Coeff_0]
  Constant2/1 -> [Filter_Coeff_1]
  Derivative/1 -> Scope3/2
  use true/1 -> [Use_true]

== system Simulink_MPC_Main/SOLVE OCP /Subsystem1/MPC 1/Subsystem4 ==
  In1 : Inport
  MATLAB Function8 : MATLAB Function  TreatAsAtomicUnit=on
  Scope9 : Scope
  To Workspace8 : ToWorkspace  VariableName=PAyload_mpc  SaveFormat=Structure With Time  SampleTime=-1
  wires:
  MATLAB Function8/1(first_elemt_traj) -> Scope9/1
  In1/1 -> To Workspace8/1, MATLAB Function8/1(traj)

== system Simulink_MPC_Main/SOLVE OCP /Subsystem4/MPC 1/Subsystem4 ==
  In1 : Inport
  MATLAB Function8 : MATLAB Function  TreatAsAtomicUnit=on
  Scope9 : Scope
  To Workspace8 : ToWorkspace  VariableName=PAyload_mpc  SaveFormat=Structure With Time  SampleTime=-1
  wires:
  MATLAB Function8/1(first_elemt_traj) -> Scope9/1
  In1/1 -> To Workspace8/1, MATLAB Function8/1(traj)

== system Simulink_MPC_Main/SOLVE OCP /Subsystem5/MPC 1/Subsystem4 ==
  In1 : Inport
  MATLAB Function8 : MATLAB Function  TreatAsAtomicUnit=on
  Scope9 : Scope
  To Workspace8 : ToWorkspace  VariableName=PAyload_mpc  SaveFormat=Structure With Time  SampleTime=-1
  wires:
  MATLAB Function8/1(first_elemt_traj) -> Scope9/1
  In1/1 -> To Workspace8/1, MATLAB Function8/1(traj)

== system Simulink_MPC_Main/Subsystem1/Subsystem/Subsystem5/Subsystem ==
  u : Inport
  MATLAB Function11 : MATLAB Function  TreatAsAtomicUnit=on
  MatrixMultiply : Product  Multiplication=Matrix(*)
  Out1 : Outport
  wires:
  [Filter_Coeff_0] -> MatrixMultiply/2
  MATLAB Function11/1(y) -> MatrixMultiply/1
  MatrixMultiply/1 -> Out1/1
  u/1 -> MATLAB Function11/1(u)
  [Initial_MAtrix_Buffer] -> MATLAB Function11/2(Initial_Buffer)

== system Simulink_MPC_Main/Subsystem1/Subsystem/Subsystem5/Subsystem1 ==
  u : Inport
  MATLAB Function11 : MATLAB Function  TreatAsAtomicUnit=on
  MatrixMultiply : Product  Multiplication=Matrix(*)
  Out1 : Outport
  wires:
  [Filter_Coeff_0] -> MatrixMultiply/2
  MATLAB Function11/1(y) -> MatrixMultiply/1
  MatrixMultiply/1 -> Out1/1
  u/1 -> MATLAB Function11/1(u)
  [Initial_MAtrix_Buffer] -> MATLAB Function11/2(Initial_Buffer)

== system Simulink_MPC_Main/Subsystem1/Subsystem/Subsystem5/Subsystem10 ==
  u : Inport
  MATLAB Function11 : MATLAB Function  TreatAsAtomicUnit=on
  MatrixMultiply : Product  Multiplication=Matrix(*)
  Out1 : Outport
  wires:
  [Filter_Coeff_1] -> MatrixMultiply/2
  MATLAB Function11/1(y) -> MatrixMultiply/1
  MatrixMultiply/1 -> Out1/1
  u/1 -> MATLAB Function11/1(u)
  [Initial_MAtrix_Buffer] -> MATLAB Function11/2(Initial_Buffer)

== system Simulink_MPC_Main/Subsystem1/Subsystem/Subsystem5/Subsystem11 ==
  u : Inport
  MATLAB Function11 : MATLAB Function  TreatAsAtomicUnit=on
  MatrixMultiply : Product  Multiplication=Matrix(*)
  Out1 : Outport
  wires:
  [Filter_Coeff_1] -> MatrixMultiply/2
  MATLAB Function11/1(y) -> MatrixMultiply/1
  MatrixMultiply/1 -> Out1/1
  u/1 -> MATLAB Function11/1(u)
  [Initial_MAtrix_Buffer] -> MATLAB Function11/2(Initial_Buffer)

== system Simulink_MPC_Main/Subsystem1/Subsystem/Subsystem5/Subsystem12 ==
  u : Inport
  MATLAB Function11 : MATLAB Function  TreatAsAtomicUnit=on
  MatrixMultiply : Product  Multiplication=Matrix(*)
  Out1 : Outport
  wires:
  [Filter_Coeff_1] -> MatrixMultiply/2
  MATLAB Function11/1(y) -> MatrixMultiply/1
  MatrixMultiply/1 -> Out1/1
  u/1 -> MATLAB Function11/1(u)
  [Initial_MAtrix_Buffer] -> MATLAB Function11/2(Initial_Buffer)

== system Simulink_MPC_Main/Subsystem1/Subsystem/Subsystem5/Subsystem13 ==
  u : Inport
  MATLAB Function11 : MATLAB Function  TreatAsAtomicUnit=on
  MatrixMultiply : Product  Multiplication=Matrix(*)
  Out1 : Outport
  wires:
  [Filter_Coeff_1] -> MatrixMultiply/2
  MATLAB Function11/1(y) -> MatrixMultiply/1
  MatrixMultiply/1 -> Out1/1
  u/1 -> MATLAB Function11/1(u)
  [Initial_MAtrix_Buffer] -> MATLAB Function11/2(Initial_Buffer)

== system Simulink_MPC_Main/Subsystem1/Subsystem/Subsystem5/Subsystem14 ==
  u : Inport
  MATLAB Function11 : MATLAB Function  TreatAsAtomicUnit=on
  MatrixMultiply : Product  Multiplication=Matrix(*)
  Out1 : Outport
  wires:
  [Filter_Coeff_1] -> MatrixMultiply/2
  MATLAB Function11/1(y) -> MatrixMultiply/1
  MatrixMultiply/1 -> Out1/1
  u/1 -> MATLAB Function11/1(u)
  [Initial_MAtrix_Buffer] -> MATLAB Function11/2(Initial_Buffer)

== system Simulink_MPC_Main/Subsystem1/Subsystem/Subsystem5/Subsystem2 ==
  u : Inport
  MATLAB Function11 : MATLAB Function  TreatAsAtomicUnit=on
  MatrixMultiply : Product  Multiplication=Matrix(*)
  Out1 : Outport
  wires:
  [Filter_Coeff_0] -> MatrixMultiply/2
  MATLAB Function11/1(y) -> MatrixMultiply/1
  MatrixMultiply/1 -> Out1/1
  u/1 -> MATLAB Function11/1(u)
  [Initial_MAtrix_Buffer] -> MATLAB Function11/2(Initial_Buffer)

== system Simulink_MPC_Main/Subsystem1/Subsystem/Subsystem5/Subsystem3 ==
  u : Inport
  MATLAB Function11 : MATLAB Function  TreatAsAtomicUnit=on
  MatrixMultiply : Product  Multiplication=Matrix(*)
  Out1 : Outport
  wires:
  [Filter_Coeff_0] -> MatrixMultiply/2
  MATLAB Function11/1(y) -> MatrixMultiply/1
  MatrixMultiply/1 -> Out1/1
  u/1 -> MATLAB Function11/1(u)
  [Initial_MAtrix_Buffer] -> MATLAB Function11/2(Initial_Buffer)

== system Simulink_MPC_Main/Subsystem1/Subsystem/Subsystem5/Subsystem4 ==
  u : Inport
  MATLAB Function11 : MATLAB Function  TreatAsAtomicUnit=on
  MatrixMultiply : Product  Multiplication=Matrix(*)
  Out1 : Outport
  wires:
  [Filter_Coeff_0] -> MatrixMultiply/2
  MATLAB Function11/1(y) -> MatrixMultiply/1
  MatrixMultiply/1 -> Out1/1
  u/1 -> MATLAB Function11/1(u)
  [Initial_MAtrix_Buffer] -> MATLAB Function11/2(Initial_Buffer)

== system Simulink_MPC_Main/Subsystem1/Subsystem/Subsystem5/Subsystem5 ==
  u : Inport
  Discrete Filter Coefficents : Constant  Value=|
      | [1.574208515729901059e+01
      | 1.586094721714563072e+01
      | -5.994995630757394833e-01
      | -9.191365250349250005e+00
      | -1.170290325508502960e+01
      | -9.922366987693955309e+00
      | -5.638009858585491862e+00
      | -6.380852781707303523e-01
      | 3.289153343139662233e+00
      | 4.355452594936194188e+00
      | 7.725590668082207291e-01
      | -2.327967186368518515e+00]'
  MATLAB Function11 : MATLAB Function  TreatAsAtomicUnit=on
  MatrixMultiply : Product  Multiplication=Matrix(*)
  X_Vel : Outport
  wires:
  Discrete Filter Coefficents/1 -> MatrixMultiply/2
  MATLAB Function11/1(y) -> MatrixMultiply/1
  MatrixMultiply/1 -> X_Vel/1
  u/1 -> MATLAB Function11/1(u)

== system Simulink_MPC_Main/Subsystem1/Subsystem/Subsystem5/Subsystem6 ==
  u : Inport
  Discrete Filter Coefficents : Constant  Value=|
      | [1.574208515729901059e+01
      | 1.586094721714563072e+01
      | -5.994995630757394833e-01
      | -9.191365250349250005e+00
      | -1.170290325508502960e+01
      | -9.922366987693955309e+00
      | -5.638009858585491862e+00
      | -6.380852781707303523e-01
      | 3.289153343139662233e+00
      | 4.355452594936194188e+00
      | 7.725590668082207291e-01
      | -2.327967186368518515e+00]'
  MATLAB Function11 : MATLAB Function  TreatAsAtomicUnit=on
  MatrixMultiply : Product  Multiplication=Matrix(*)
  X_Vel1 : Outport
  wires:
  Discrete Filter Coefficents/1 -> MatrixMultiply/2
  MATLAB Function11/1(y) -> MatrixMultiply/1
  MatrixMultiply/1 -> X_Vel1/1
  u/1 -> MATLAB Function11/1(u)

== system Simulink_MPC_Main/Subsystem1/Subsystem/Subsystem5/Subsystem7 ==
  u : Inport
  Derivative : Derivative
  Discrete Filter Coefficents : Constant  Value=|
      | [1.574208515729901059e+01
      | 1.586094721714563072e+01
      | -5.994995630757394833e-01
      | -9.191365250349250005e+00
      | -1.170290325508502960e+01
      | -9.922366987693955309e+00
      | -5.638009858585491862e+00
      | -6.380852781707303523e-01
      | 3.289153343139662233e+00
      | 4.355452594936194188e+00
      | 7.725590668082207291e-01
      | -2.327967186368518515e+00]'
  MATLAB Function11 : MATLAB Function  TreatAsAtomicUnit=on
  MatrixMultiply : Product  Multiplication=Matrix(*)
  Scope : Scope  NumInputPorts=2
  Out1 : Outport
  wires:
  Discrete Filter Coefficents/1 -> MatrixMultiply/2
  MATLAB Function11/1(y) -> MatrixMultiply/1
  MatrixMultiply/1 -> Scope/1, Out1/1
  u/1 -> Derivative/1, MATLAB Function11/1(u)
  Derivative/1 -> Scope/2

== system Simulink_MPC_Main/Subsystem1/Subsystem/Subsystem5/Subsystem8 ==
  u : Inport
  Discrete Filter Coefficents : Constant  Value=|
      | [1.574208515729901059e+01
      | 1.586094721714563072e+01
      | -5.994995630757394833e-01
      | -9.191365250349250005e+00
      | -1.170290325508502960e+01
      | -9.922366987693955309e+00
      | -5.638009858585491862e+00
      | -6.380852781707303523e-01
      | 3.289153343139662233e+00
      | 4.355452594936194188e+00
      | 7.725590668082207291e-01
      | -2.327967186368518515e+00]'
  MATLAB Function11 : MATLAB Function  TreatAsAtomicUnit=on
  MatrixMultiply : Product  Multiplication=Matrix(*)
  Out1 : Outport
  wires:
  Discrete Filter Coefficents/1 -> MatrixMultiply/2
  MATLAB Function11/1(y) -> MatrixMultiply/1
  MatrixMultiply/1 -> Out1/1
  u/1 -> MATLAB Function11/1(u)

== system Simulink_MPC_Main/Subsystem1/Subsystem/Subsystem5/Subsystem9 ==
  u : Inport
  Derivative : Derivative
  Discrete Filter Coefficents : Constant  Value=|
      | [1.574208515729901059e+01
      | 1.586094721714563072e+01
      | -5.994995630757394833e-01
      | -9.191365250349250005e+00
      | -1.170290325508502960e+01
      | -9.922366987693955309e+00
      | -5.638009858585491862e+00
      | -6.380852781707303523e-01
      | 3.289153343139662233e+00
      | 4.355452594936194188e+00
      | 7.725590668082207291e-01
      | -2.327967186368518515e+00]'
  MATLAB Function11 : MATLAB Function  TreatAsAtomicUnit=on
  MatrixMultiply : Product  Multiplication=Matrix(*)
  Scope : Scope  NumInputPorts=2
  Out1 : Outport
  wires:
  Discrete Filter Coefficents/1 -> MatrixMultiply/2
  MATLAB Function11/1(y) -> MatrixMultiply/1
  Derivative/1 -> Scope/2
  u/1 -> Derivative/1, MATLAB Function11/1(u)
  MatrixMultiply/1 -> Scope/1, Out1/1

== matlab function Simulink_MPC_Main/Subsystem1/Subsystem/Subsystem5/MATLAB Function ==
  data: Initial_MAtrix output
function Initial_MAtrix = Immutable_Constant_Matrix()

Initial_MAtrix = ones(10,1);

== matlab function Simulink_MPC_Main/Subsystem1/Subsystem/Limit Input/MATLAB Function5 ==
  data: PWL input; PWL_Limit output; Position input; epsilon input
function PWL_Limit = fcn(PWL,Position,epsilon)

if (PWL < 0) && (Position-epsilon <= 0)
 PWL_Limit = 0;
else if (PWL > 0) && (Position+epsilon >= 0.49876)
     PWL_Limit = 0    ;
else
 PWL_Limit = PWL;
end
end

== matlab function Simulink_MPC_Main/Subsystem1/Subsystem/Limit Input/MATLAB Function6 ==
  data: PWL input; PWL_Limit output; Position input; epsilon input

function PWL_Limit = fcn(PWL,Position,epsilon)

if (PWL < 0) && (Position-epsilon <= 0)
 PWL_Limit = 0;
else if (PWL > 0) && (Position+epsilon >= 0.62159)
     PWL_Limit = 0    ;
else
 PWL_Limit = PWL;
end
end

== matlab function Simulink_MPC_Main/SOLVE OCP /Subsystem/Delete L ==
  data: x10 input; x_8 output
function x_8 = fcn(x10)
relevantstates = [1,2,4,5,6,7,9,10];
x_8 =x10(relevantstates);

== matlab function Simulink_MPC_Main/SOLVE OCP /Subsystem5/MPC 1/MATLAB Function ==
  data: x input; x_warm output
function x_warm = fcn(x)
x_warm = [x(:,3:end) x(:,end)];

== matlab function Simulink_MPC_Main/Subsystem1/Subsystem/Limit Input/MATLAB Function4 ==
  data: PWL input; PWL_Limit output; Position input; epsilon input
function PWL_Limit = fcn(PWL,Position,epsilon)

if (PWL < 0) && (Position-epsilon <= 0)
 PWL_Limit = 0;
else if (PWL > 0) && (Position+epsilon >= 0.55004)
     PWL_Limit = 0    ;
else
 PWL_Limit = PWL;
end
end
% 0.55004

== matlab function Simulink_MPC_Main/Subsystem1/Subsystem/Subsystem5/Subsystem/MATLAB Function11 ==
  settings: updateMethod=DISCRETE
  data: u input; y output size=[1,N_Coeff]; Initial_Buffer input
function y = CircularBuffer(u,Initial_Buffer)
%#codegen
% Function to implement a simple N element circular buffer

% Define the internal buffer variable as persistent
persistent buffer



% Initialize the buffer the first time through
if isempty(buffer)
    % Initialize the buffer
    buffer = Initial_Buffer*u;
    % buff_entrys = 1;
    buffer(1) = u;
else
    % wenn nicht leer, dann schiebe eins hoch 
    buff2 = buffer; 
    buffer = [u; buff2(1:end-1)];
end

% Output the buffer
y = buffer';

end

== matlab function Simulink_MPC_Main/SOLVE OCP /Subsystem5/MPC 1/MATLAB Function1 ==
  data: lam_g input; lam_g_warm output
function lam_g_warm = fcn(lam_g)
lam_g_warm = lam_g;

== matlab function Simulink_MPC_Main/SOLVE OCP /Subsystem5/MPC 1/MATLAB Function2 ==
  data: u input; u_warm output size=DimU
function u_warm = fcn(u)

u_warm = [u(:,2:end) u(:,end)];

== matlab function Simulink_MPC_Main/SOLVE OCP /Subsystem5/MATLAB Function3 ==
  data: u input; u_plant output size=[1,1]; x input; x_new output
function [u_plant,x_new] = fcn(u,x)

x_new = x(:,2);
u_plant = u(:,1);

== matlab function Simulink_MPC_Main/Nonlinear Model/MATLAB Function4 ==
  data: x_in input; PWM input; x_end output; SampleTime input
function x_end   = Integrate_rk4(x_in, PWM,SampleTime)

% X_PWM_Simtime = PWM(1,:);
% Y_PWM_Simtime = PWM(2,:);
% Z_PWM_Simtime = PWM(3,:);
dt =  0.0002; % Time step for RK4 integration
% nSteps = 451;
nSteps = SampleTime/dt +1;
% l0 = 0.1712;
params = struct;
% Initialize output matrix for the RK4 results
% Apply coordinate transform to fit model
% x = [x_in(1) x_in(2) x_in(3)+l0  x_in(4) x_in(5) x_in(6) (x_in(7)) x_in(8) x_in(9) x_in(10)]; % Initial state
x = x_in';
% rk4Results = zeros(nSteps, length(x));
% rk4Results(1, :) = x_in'; % Initial state

for i = 1:nSteps-1
    % Current input
    u = [PWM(1) PWM(2) 0];
    % RK4 Integration
    k1 = crane3DModel_derivation(x, u);
    k2 = crane3DModel_derivation(x + 0.5*dt*k1, u);
    k3 = crane3DModel_derivation(x + 0.5*dt*k2, u);
    k4 = crane3DModel_derivation(x + dt*k3, u);
    
    x = x + dt*(k1 + 2*k2 + 2*k3 + k4)/6;
    % rk4Results(i+1, :) = [x(1), x(2), x(3)-l0,(x(4)), x(5) ,x(6), x(7), x(8), x(9), x(10)];
  % rk4Results(i+1, :) = x;

end
x_end = x;
end

== matlab function Simulink_MPC_Main/Subsystem1/Subsystem/Subsystem5/Subsystem5/MATLAB Function11 ==
  settings: updateMethod=DISCRETE  sampleTime=0.01
  data: u input; y output size=1
function y = CircularBuffer(u)
%#codegen
% Function to implement a simple N element circular buffer

% Define the internal buffer variable as persistent
persistent buffer

N = 12;

% Initialize the buffer the first time through
if isempty(buffer)
    % Initialize the buffer
    buffer = zeros(N,1);
    % buff_entrys = 1;
    buffer(1) = u;
else
    % wenn nicht leer, dann schiebe eins hoch 
    buff2 = buffer; 
    buffer = [u; buff2(1:N-1)];
end

% Output the buffer
y = buffer';

end

== matlab function Simulink_MPC_Main/Subsystem1/Subsystem/Subsystem5/Subsystem6/MATLAB Function11 ==
  settings: updateMethod=DISCRETE  sampleTime=0.01
  data: u input; y output
function y = CircularBuffer(u)
%#codegen
% Function to implement a simple N element circular buffer

% Define the internal buffer variable as persistent
persistent buffer

N = 12;

% Initialize the buffer the first time through
if isempty(buffer)
    % Initialize the buffer
    buffer = zeros(N,1);
    % buff_entrys = 1;
    buffer(1) = u;
else
    % wenn nicht leer, dann schiebe eins hoch 
    buff2 = buffer; 
    buffer = [u; buff2(1:N-1)];
end

% Output the buffer
y = buffer';

end

== matlab function Simulink_MPC_Main/Subsystem1/Subsystem/Subsystem5/Subsystem7/MATLAB Function11 ==
  settings: updateMethod=DISCRETE  sampleTime=0.01
  data: u input; y output
function y = CircularBuffer(u)
%#codegen
% Function to implement a simple N element circular buffer

% Define the internal buffer variable as persistent
persistent buffer

N = 12;

% Initialize the buffer the first time through
if isempty(buffer)
    % Initialize the buffer
    buffer = zeros(N,1);
    % buff_entrys = 1;
    buffer(1) = u;
else
    % wenn nicht leer, dann schiebe eins hoch 
    buff2 = buffer; 
    buffer = [u; buff2(1:N-1)];
end

% Output the buffer
y = buffer';

end

== matlab function Simulink_MPC_Main/Subsystem1/Subsystem/Subsystem5/Subsystem8/MATLAB Function11 ==
  settings: updateMethod=DISCRETE  sampleTime=0.01
  data: u input; y output
function y = CircularBuffer(u)
%#codegen
% Function to implement a simple N element circular buffer

% Define the internal buffer variable as persistent
persistent buffer

N = 12;

% Initialize the buffer the first time through
if isempty(buffer)
    % Initialize the buffer
    buffer = zeros(N,1);
    % buff_entrys = 1;
    buffer(1) = u;
else
    % wenn nicht leer, dann schiebe eins hoch 
    buff2 = buffer; 
    buffer = [u; buff2(1:N-1)];
end

% Output the buffer
y = buffer';

end

== matlab function Simulink_MPC_Main/Subsystem1/Subsystem/Subsystem5/Subsystem9/MATLAB Function11 ==
  settings: updateMethod=DISCRETE  sampleTime=0.01
  data: u input; y output
function y = CircularBuffer(u)
%#codegen
% Function to implement a simple N element circular buffer

% Define the internal buffer variable as persistent
persistent buffer

N = 12;

% Initialize the buffer the first time through
if isempty(buffer)
    % Initialize the buffer
    buffer = zeros(N,1);
    % buff_entrys = 1;
    buffer(1) = u;
else
    % wenn nicht leer, dann schiebe eins hoch 
    buff2 = buffer; 
    buffer = [u; buff2(1:N-1)];
end

% Output the buffer
y = buffer';

end

== matlab function Simulink_MPC_Main/Subsystem3/dry_friction_compensation ==
  data: x input; u input; u_compensated output
function u_compensated = fcn(x,u)
% u_compensated = u+[-0.1576*sign(100*x(5)); -0.1232*sign(100*x(6))];
% u_compensated = u+[-0.1576*sign(100*u(1)); -0.1232*sign(100*u(2))];
u_compensated = zeros(2,1);
if abs(u(1)) > 0.01
u_compensated(1) = u(1) +  0.1576*tanh(200*x(6));
% u_compensated(1) = u(1) +  0.006*tanh(200*x(6));
end
if abs(u(2)) > 0.01
u_compensated(2) = u(2) +  0.1232*tanh(200*x(7));
end
% u_compensated = u + [0.1576*tanh(2000*x(6)); 0.1232*tanh(2000*x(7))];

== matlab function Simulink_MPC_Main/Nonlinear Model/MATLAB Function3 ==
  data: x input; current output
function current = fcn(x)
current = [x(:,1)];

== matlab function Simulink_MPC_Main/Subsystem1/Subsystem/MATLAB Function ==
  data: Positions output size=[1, 5]; PWM_X input; PWM_Y input; PWM_Z input; Time output
function [Positions,Time]  = Driver(PWM_X, PWM_Y, PWM_Z)

persistent starttime


% Input = [0.1 0.1 0.1];
Positions = [0 0 0 0 0];
PWM = [0 0 0];
Time1 = 0;
[Positions Time1] = UpdateBoard([PWM_X, PWM_Y, PWM_Z]);
if isempty(starttime)
    starttime = Time1;
end
Time = (Time1 - starttime)/1000;

% Positions = [0,0,0,0,0];
% % Positions = getEncoderCounter();
% Positions = Positions';
end

== matlab function Simulink_MPC_Main/SOLVE OCP /Nonlinear Model1/MATLAB Function ==
  data: x input; x_bound output
function x_bound = fcn(x)
x_bound = x;
if x_bound(1) < 0.01
    x_bound(1) = 0.01;
end
if x_bound(1) > 0.49
    x_bound(1) = 0.49;
end
if x_bound(2) < 0.01
    x_bound(2) = 0.01;
end
if x_bound(2) > 0.59
    x_bound(2) = 0.59;
end

== matlab function Simulink_MPC_Main/SOLVE OCP /Subsystem4/MATLAB Function3 ==
  data: u input; u_plant output size=[1,1]; x input
function u_plant = fcn(u,x)

x_new = x(:,2);
u_plant = u(:,1);

== matlab function Simulink_MPC_Main/SOLVE OCP /Subsystem5/MPC 1/Subsystem4/MATLAB Function8 ==
  data: traj input; first_elemt_traj output
function first_elemt_traj = getfirstelement(traj)

first_elemt_traj = traj(:,1);

== matlab function Simulink_MPC_Main/SOLVE OCP /Subsystem4/MPC 1/MATLAB Function ==
  data: x input; x_warm output
function x_warm = fcn(x)
x_warm = [x(:,3:end) x(:,end)];

== matlab function Simulink_MPC_Main/SOLVE OCP /Subsystem/MATLAB Function10 ==
  data: x_18 input; x_X output; x_Y output
function [x_X,x_Y] = add_int(x_18)
x_X = zeros(4,1);
x_Y = zeros(4,1);
x_X(1) = x_18(1);
x_Y(1) = x_18(2);
x_X(2) = x_18(3);
x_Y(2) = x_18(4);
x_X(3) = x_18(5);
x_Y(3) = x_18(6);
x_X(4) = x_18(7);
x_Y(4) = x_18(8);

== matlab function Simulink_MPC_Main/SOLVE OCP /Subsystem4/MPC 1/MATLAB Function1 ==
  data: lam_g input; lam_g_warm output
function lam_g_warm = fcn(lam_g)
lam_g_warm = lam_g;
